simulink model "ejercicio3"  (R2025b)
settings: Solver=VariableStepAuto  StartTime=0.0  StopTime=10.0  RelTol=1e-3
libraries: fuzblock x1
settings Model: Creator=chenfu  LastModifiedBy=chenfu

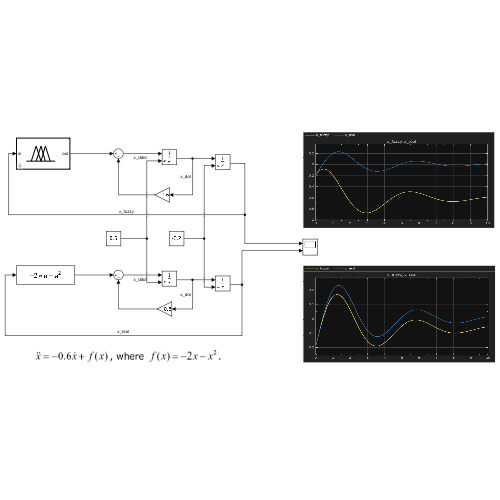
[thumbnail: Simulink's stored preview of the top-level diagram]
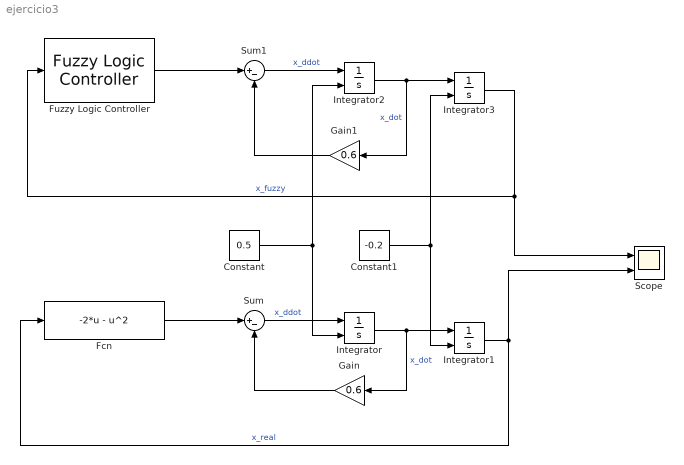
== system ejercicio3 ==
  Constant : Constant  Value=0.5
  Constant1 : Constant  Value=-0.2
  Fcn : Fcn  Expr=-2*u - u^2
  Fuzzy Logic Controller : fuzblock/Fuzzy Logic  Controller  FIS=fismat1  OutputSampleNumber=101  DataType=double  UseLookupTable=off  NumBreakpoints=10  FuzzifiedInputs=off  RuleFiringStrengths=off  RuleOutputs=off  AggregatedOutputs=off  SimulateUsing=Interpreted execution  OutOfRangeInputValueMessage=warning  NoRuleFiredMessage=warning  EmptyOutputFuzzySetMessage=warning
  Gain : Gain  Gain=0.6
  Gain1 : Gain  Gain=0.6
  Integrator{,1..3} (4 alike) : Integrator  InitialConditionSource=external
  Scope : Scope  NumInputPorts=2
      settings: ActiveDisplayYMinimum=-1.0168526420319413  ActiveDisplayYMaximum=0.37038562378010342
  Sum : Sum  Inputs=|+-
  Sum1 : Sum  Inputs=|+-
  wires:
  Fcn/1 -> Sum/1
  Sum/1 -> Integrator/1  "x_ddot"
  Integrator/1 -> Integrator1/1, Gain/1  "x_dot"
  Gain/1 -> Sum/2
  Integrator1/1 -> Scope/2, Fcn/1  "x_real"
  Fuzzy Logic Controller/1 -> Sum1/1
  Integrator2/1 -> Integrator3/1, Gain1/1  "x_dot"
  Gain1/1 -> Sum1/2
  Integrator3/1 -> Scope/1, Fuzzy Logic Controller/1  "x_fuzzy"
  Sum1/1 -> Integrator2/1  "x_ddot"
  Constant/1 -> Integrator2/2, Integrator/2
  Constant1/1 -> Integrator3/2, Integrator1/2
